simulink model "SRS_AverageSlopeTest"  (R2023b)
settings: Solver=FixedStepAuto  StartTime=0.0  StopTime=150  FixedStep=0.001  MaxStep=0.001  RelTol=1e-3
libraries: simulink x6, Solver_SF x1
settings Model: DataTypeOverride=Double  MinMaxOverflowLogging=ForceOff  Creator=황수빈  LastModifiedBy=황수빈

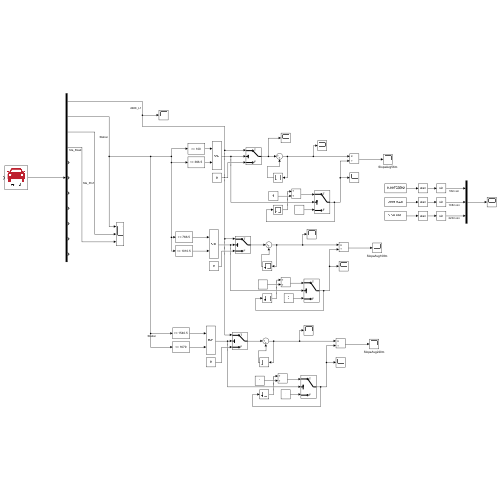
[thumbnail: Simulink's stored preview of the top-level diagram]
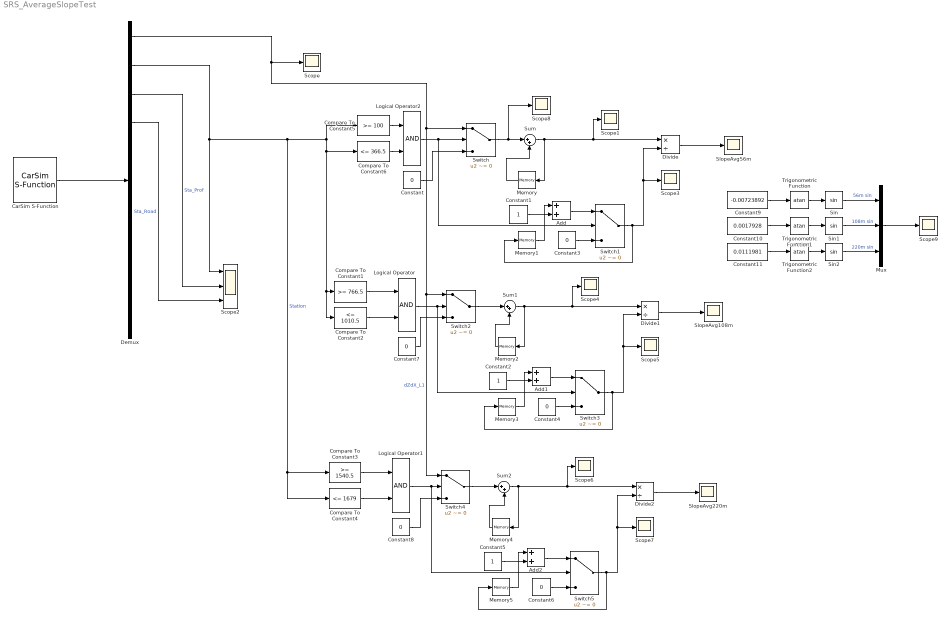
== system SRS_AverageSlopeTest ==
  Add : Sum
  Add1 : Sum
  Add2 : Sum
  CarSim S-Function : Solver_SF/CarSim S-Function  Priority=1  SIMFILE=simfile.sim  Run_RTs=off  vs_state_ind=Run  StopMode_ind=Vehicle Model
  Compare To Constant1 : simulink/Logic and Bit Operations/Compare To Constant  relop=>=  const=766.5  OutDataTypeStr=boolean
  Compare To Constant2 : simulink/Logic and Bit Operations/Compare To Constant  relop=<=  const=1010.5  OutDataTypeStr=boolean
  Compare To Constant3 : simulink/Logic and Bit Operations/Compare To Constant  relop=>=  const=1540.5  OutDataTypeStr=boolean
  Compare To Constant4 : simulink/Logic and Bit Operations/Compare To Constant  relop=<=  const=1679  OutDataTypeStr=boolean
  Compare To Constant5 : simulink/Logic and Bit Operations/Compare To Constant  relop=>=  const=100  OutDataTypeStr=boolean
  Compare To Constant6 : simulink/Logic and Bit Operations/Compare To Constant  relop=<=  const=366.5  OutDataTypeStr=boolean
  Constant{,3..4,6..8} (6 alike) : Constant  Value=0
  Constant1 : Constant
  Constant10 : Constant  Value=0.0017928
  Constant11 : Constant  Value=0.0111981
  Constant2 : Constant
  Constant5 : Constant
  Constant9 : Constant  Value=-0.00723892
  Demux : Demux  Outputs=11
  Divide : Product  Inputs=*/
  Divide1 : Product  Inputs=*/
  Divide2 : Product  Inputs=*/
  Logical Operator : Logic  AllPortsSameDT=off  OutDataTypeStr=boolean
  Logical Operator1 : Logic  AllPortsSameDT=off  OutDataTypeStr=boolean
  Logical Operator2 : Logic  AllPortsSameDT=off  OutDataTypeStr=boolean
  Memory{,1..5} (6 alike) : Memory
  Mux : Mux  Inputs=3
  Scope{,1,3..9} (9 alike) : Scope
  Scope2 : Scope  NumInputPorts=3
  Sin : Trigonometry
  Sin1 : Trigonometry
  Sin2 : Trigonometry
  SlopeAvg108m : Scope
  SlopeAvg220m : Scope
  SlopeAvg56m : Scope
  Sum : Sum  Inputs=|++
  Sum1 : Sum  Inputs=|++
  Sum2 : Sum  Inputs=|++
  Switch{,1..5} (6 alike) : Switch  Criteria=u2 ~= 0  SaturateOnIntegerOverflow=off  InputSameDT=off
  Trigonometric Function : Trigonometry  Operator=atan
  Trigonometric Function1 : Trigonometry  Operator=atan
  Trigonometric Function2 : Trigonometry  Operator=atan
  wires:
  CarSim S-Function/1 -> Demux/1
  Demux/1 -> Switch2/1, Switch4/1, Switch/1, Scope/1  "dZdX_L1"
  Demux/3 -> Scope2/2  "Sta_Prof"
  Demux/4 -> Scope2/3  "Sta_Road"
  Logical Operator2/1 -> Switch1/2, Switch/2
  Switch/1 -> Scope8/1, Sum/1
  Memory/1 -> Sum/2
  Sum/1 -> Scope1/1, Divide/1, Memory/1
  Constant1/1 -> Add/2
  Add/1 -> Switch1/1
  Memory1/1 -> Add/1
  Switch1/1 -> Memory1/1, Scope3/1, Divide/2
  Divide/1 -> SlopeAvg56m/1
  Logical Operator/1 -> Switch3/2, Switch2/2
  Compare To Constant1/1 -> Logical Operator/1
  Compare To Constant2/1 -> Logical Operator/2
  Switch3/1 -> Memory3/1, Scope5/1, Divide1/2
  Add1/1 -> Switch3/1
  Divide1/1 -> SlopeAvg108m/1
  Constant2/1 -> Add1/2
  Memory3/1 -> Add1/1
  Memory2/1 -> Sum1/2
  Sum1/1 -> Scope4/1, Divide1/1, Memory2/1
  Switch2/1 -> Sum1/1
  Constant3/1 -> Switch1/3
  Constant4/1 -> Switch3/3
  Divide2/1 -> SlopeAvg220m/1
  Sum2/1 -> Scope6/1, Divide2/1, Memory4/1
  Memory5/1 -> Add2/1
  Memory4/1 -> Sum2/2
  Switch5/1 -> Memory5/1, Scope7/1, Divide2/2
  Constant5/1 -> Add2/2
  Constant6/1 -> Switch5/3
  Logical Operator1/1 -> Switch5/2, Switch4/2
  Constant/1 -> Switch/3
  Compare To Constant3/1 -> Logical Operator1/1
  Demux/2 -> Compare To Constant6/1, Compare To Constant1/1, Compare To Constant2/1, Compare To Constant5/1, Compare To Constant3/1, Compare To Constant4/1, Scope2/1  "Station"
  Compare To Constant4/1 -> Logical Operator1/2
  Add2/1 -> Switch5/1
  Switch4/1 -> Sum2/1
  Constant7/1 -> Switch2/3
  Constant8/1 -> Switch4/3
  Compare To Constant5/1 -> Logical Operator2/1
  Compare To Constant6/1 -> Logical Operator2/2
  Constant9/1 -> Trigonometric Function/1
  Trigonometric Function/1 -> Sin/1
  Sin/1 -> Mux/1  "56m sin"
  Constant10/1 -> Trigonometric Function1/1
  Trigonometric Function1/1 -> Sin1/1
  Sin1/1 -> Mux/2  "108m sin"
  Constant11/1 -> Trigonometric Function2/1
  Trigonometric Function2/1 -> Sin2/1
  Sin2/1 -> Mux/3  "220m sin"
  Mux/1 -> Scope9/1
